simulink model "pendule_inv_echant_etu"  (R2022a)
settings: Solver=VariableStepAuto  StartTime=0.0  StopTime=10.0  RelTol=1e-3
values from neighbouring files (symbols this model uses):
  g = 9.81    [simu_pendule_inv_capteur_etu.m]    (also in simu_pendule_inv_etu.m)
  K = [10 1]    [simu_pendule_inv_capteur_etu.m]    (also in simu_pendule_inv_etu.m)
  l = 10    [simu_pendule_inv_capteur_etu.m]    (also in simu_pendule_inv_etu.m)
  ue = 0    [simu_pendule_inv_capteur_etu.m]    (also in simu_pendule_inv_etu.m)
  x0 = [pi/20 0]'    [simu_pendule_inv_capteur_etu.m]    (also in simu_pendule_inv_etu.m)
  xe = [0 0]'    [simu_pendule_inv_capteur_etu.m]    (also in simu_pendule_inv_etu.m)
undefined symbols (not defined in the file or in its folder): delta_t, DiscIntNeverNeededParam
settings Model: Creator=lthietar  LastModifiedBy=lthietar

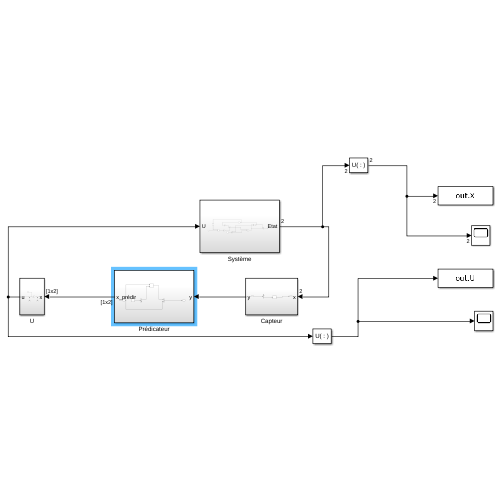
[thumbnail: Simulink's stored preview of the top-level diagram]
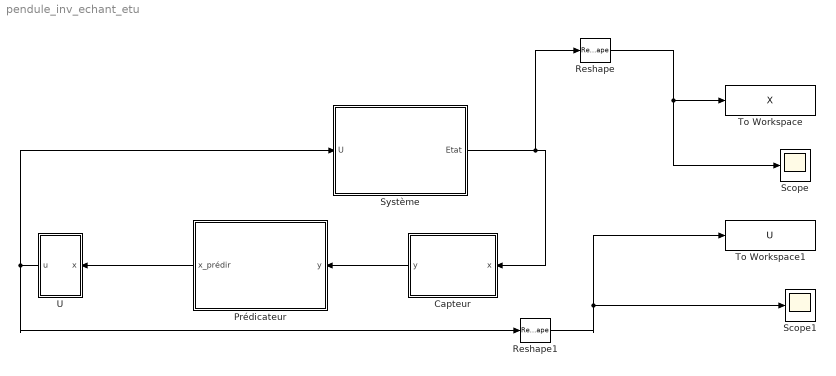
== system pendule_inv_echant_etu ==
  Capteur : Subsystem
  Prédicateur : Subsystem
  Reshape : Reshape
  Reshape1 : Reshape
  Scope : Scope
  Scope1 : Scope
  Système : Subsystem
  To Workspace : ToWorkspace  VariableName=X  SaveFormat=Timeseries  SampleTime=-1
  To Workspace1 : ToWorkspace  VariableName=U  SaveFormat=Timeseries  SampleTime=-1
  U : Subsystem
  wires:
  U/1(u) -> Système/1(U), Reshape1/1
  Capteur/1(y) -> Prédicateur/1(y)
  Prédicateur/1(x_prédir) -> U/1(x)
  Système/1(Etat) -> Capteur/1(x), Reshape/1
  Reshape/1 -> Scope/1, To Workspace/1
  Reshape1/1 -> To Workspace1/1, Scope1/1

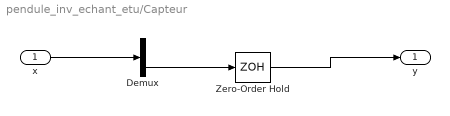
== system pendule_inv_echant_etu/Capteur ==
  x : Inport
  Demux : Demux  Outputs=2
  Zero-Order Hold : ZeroOrderHold  SampleTime=-1
  y : Outport
  wires:
  x/1 -> Demux/1
  Demux/2 -> Zero-Order Hold/1
  Zero-Order Hold/1 -> y/1

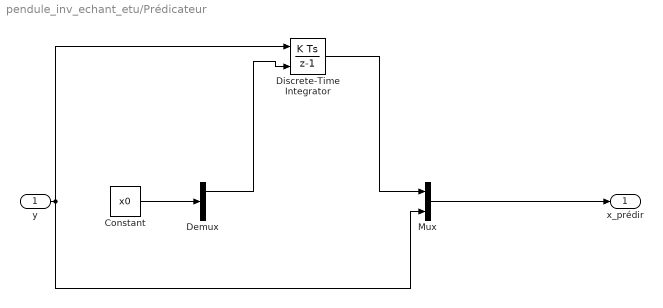
== system pendule_inv_echant_etu/Prédicateur ==
  y : Inport
  Constant : Constant  Value=x0
  Demux : Demux  Outputs=2
  Discrete-Time Integrator : DiscreteIntegrator  InitialConditionSource=external  SampleTime=delta_t  ICPrevOutput=DiscIntNeverNeededParam  ICPrevScaledInput=DiscIntNeverNeededParam
  Mux : Mux  Inputs=2
  x_prédir : Outport
  wires:
  Mux/1 -> x_prédir/1
  y/1 -> Mux/2, Discrete-Time Integrator/1
  Discrete-Time Integrator/1 -> Mux/1
  Constant/1 -> Demux/1
  Demux/1 -> Discrete-Time Integrator/2

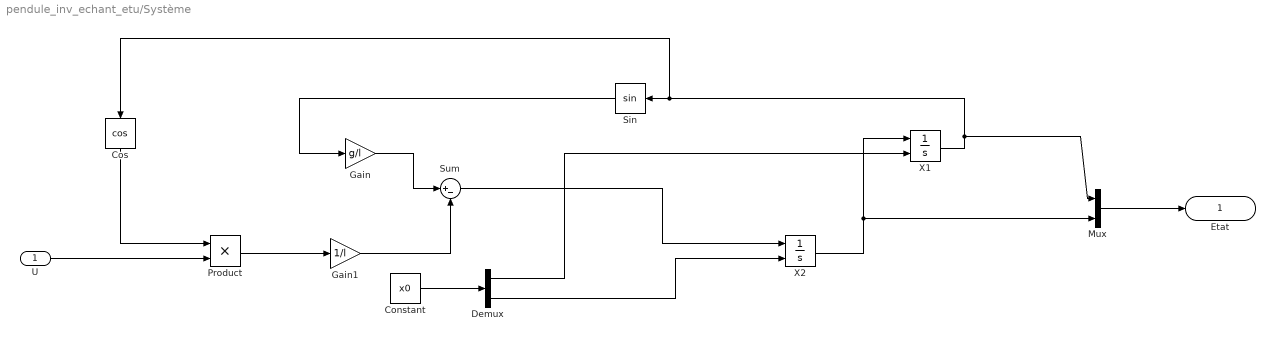
== system pendule_inv_echant_etu/Système ==
  U : Inport
  Constant : Constant  Value=x0  VectorParams1D=off
  Cos : Trigonometry  Operator=cos
  Demux : Demux  Outputs=2
  Gain : Gain  Gain=g/l
  Gain1 : Gain  Gain=1/l
  Mux : Mux  Inputs=2
  Product : Product
  Sin : Trigonometry
  Sum : Sum  Inputs=|+-
  X1 : Integrator  InitialConditionSource=external
  X2 : Integrator  InitialConditionSource=external
  Etat : Outport
  wires:
  Constant/1 -> Demux/1
  Demux/1 -> X1/2
  X2/1 -> Mux/2, X1/1
  Gain/1 -> Sum/1
  X1/1 -> Cos/1, Sin/1, Mux/1
  Sin/1 -> Gain/1
  Gain1/1 -> Sum/2
  Sum/1 -> X2/1
  Demux/2 -> X2/2
  Product/1 -> Gain1/1
  Cos/1 -> Product/1
  U/1 -> Product/2
  Mux/1 -> Etat/1

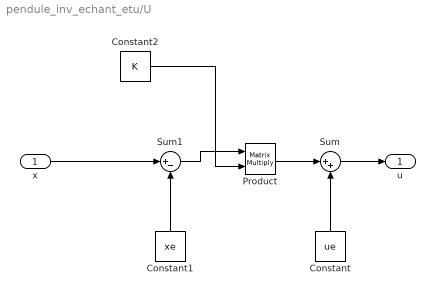
== system pendule_inv_echant_etu/U ==
  x : Inport
  Constant : Constant  Value=ue
  Constant1 : Constant  Value=xe
  Constant2 : Constant  Value=K
  Product : Product  Multiplication=Matrix(*)
  Sum : Sum  Inputs=|++
  Sum1 : Sum  Inputs=|+-
  u : Outport
  wires:
  Constant/1 -> Sum/2
  Sum/1 -> u/1
  Constant1/1 -> Sum1/2
  x/1 -> Sum1/1
  Product/1 -> Sum/1
  Sum1/1 -> Product/1
  Constant2/1 -> Product/2
